simulink model "supercontrol"  (Simulink 7.8)
settings: Solver=ode45  StartTime=0.0  StopTime=10.0  RelTol=1e-3
values from neighbouring files (symbols this model uses):
  A = [0 -23.8; 0 0]    [controllerdesign.m]
  B = [0; -23.8]    [controllerdesign.m]
  Kd = 0.1    [controllerdesign.m]
libraries: simulink x1
settings Model: Creator=pau  LastModifiedBy=pau

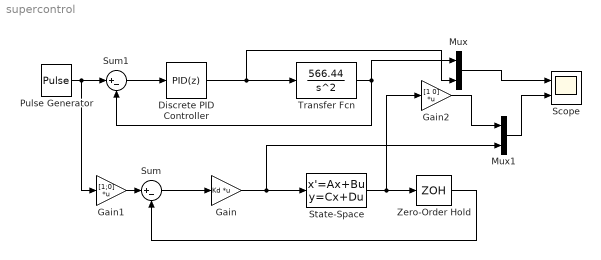
== system supercontrol ==
  Discrete PID Controller : simulink/Continuous/PID Controller  Controller=PID  TimeDomain=Discrete-time  SampleTime=0.05  IntegratorMethod=Forward Euler  FilterMethod=Forward Euler  Form=Parallel  P=0.00715782340054186  I=0.000362110080421998  D=0.0110982769773743  N=14.64502548838  InitialConditionSource=internal  InitialConditionForIntegrator=0  InitialConditionForFilter=0  ExternalReset=none  LimitOutput=off  UpperSaturationLimit=inf  LowerSaturationLimit=-inf  LinearizeAsGain=off  AntiWindupMode=none  Kb=1  TrackingMode=off  Kt=1  PParamMin=[]  PParamMax=[]  IParamMin=[]  IParamMax=[]  DParamMin=[]  DParamMax=[]  NParamMin=[]  NParamMax=[]  KbParamMin=[]  KbParamMax=[]  KtParamMin=[]  KtParamMax=[]  POutMin=[]  POutMax=[]  IOutMin=[]  IOutMax=[]  DOutMin=[]  DOutMax=[]  NOutMin=[]  NOutMax=[]  KbOutMin=[]  KbOutMax=[]  KtOutMin=[]  KtOutMax=[]  IntegratorOutMin=[]  IntegratorOutMax=[]  FilterOutMin=[]  FilterOutMax=[]  SumOutMin=[]  SumOutMax=[]  SumI1OutMin=[]  SumI1OutMax=[]  SumI2OutMin=[]  SumI2OutMax=[]  SumI3OutMin=[]  SumI3OutMax=[]  SumDOutMin=[]  SumDOutMax=[]  SaturationOutMin=[]  SaturationOutMax=[]  IntegratorContinuousStateAttributes=''  IntegratorStateMustResolveToSignalObject=off  IntegratorRTWStateStorageClass=Auto  FilterContinuousStateAttributes=''  FilterStateMustResolveToSignalObject=off  FilterRTWStateStorageClass=Auto
  Gain : Gain  Gain=Kd  Multiplication=Matrix(K*u)
  Gain1 : Gain  Gain=[1;0]  Multiplication=Matrix(K*u)
  Gain2 : Gain  Gain=[1 0]  Multiplication=Matrix(K*u)
  Mux : Mux  Inputs=2
  Mux1 : Mux  Inputs=2
  Pulse Generator : DiscretePulseGenerator  PulseType=Time based  Period=4  PulseWidth=50
  Scope : Scope  NumInputPorts=2
      settings: YMin=-5~-5  YMax=5~5
  State-Space : StateSpace  A=A  B=B  C=eye(2)  D=[0;0]
  Sum : Sum  Inputs=|+-
  Sum1 : Sum  Inputs=|+-
  Transfer Fcn : TransferFcn  Numerator=[566.44]  Denominator=[1 0 0]
  Zero-Order Hold : ZeroOrderHold  SampleTime=0.05
  wires:
  Discrete PID Controller/1 -> Transfer Fcn/1, Mux/2
  Transfer Fcn/1 -> Sum1/2, Mux/1
  Pulse Generator/1 -> Sum1/1, Gain1/1
  Sum1/1 -> Discrete PID Controller/1
  Sum/1 -> Gain/1
  Gain/1 -> State-Space/1, Mux1/2
  State-Space/1 -> Zero-Order Hold/1, Gain2/1
  Zero-Order Hold/1 -> Sum/2
  Gain1/1 -> Sum/1
  Mux/1 -> Scope/1
  Gain2/1 -> Mux1/1
  Mux1/1 -> Scope/2
